simulink model "COSIM"  (R2013b)
settings: Solver=FixedStepDiscrete  StartTime=0.0  StopTime=N  RelTol=1e-3
libraries: modelsimlib x1
settings Model: Creator=o_cotte  LastModifiedBy=o_cotte

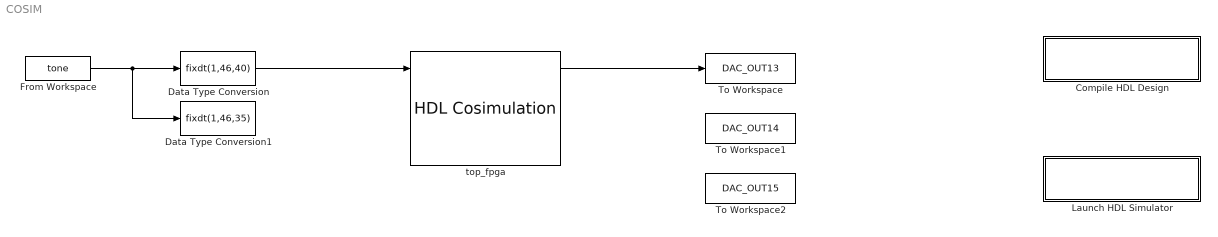
== system COSIM ==
  Compile HDL Design : Subsystem
      settings: OpenFcn=eval('compile_hdl_design_top_fpga');
      mask Display: disp(['Double-Click to' char(10) 'compile HDL files'])
  Data Type Conversion : DataTypeConversion  OutDataTypeStr=fixdt(1,46,40)
  Data Type Conversion1 : DataTypeConversion  OutDataTypeStr=fixdt(1,46,35)
  From Workspace : FromWorkspace  VariableName=tone  SampleTime=1  Interpolate=off  OutputAfterFinalValue=Cyclic repetition
  Launch HDL Simulator : Subsystem
      settings: OpenFcn=eval('launch_hdl_simulator_top_fpga');
      mask Display: disp(['Double-Click to' char(10) 'launch HDL simulator'])
  To Workspace : ToWorkspace  VariableName=DAC_OUT13  SampleTime=-1
  To Workspace1 : ToWorkspace  VariableName=DAC_OUT14  SampleTime=-1  SaveFormat=Timeseries
  To Workspace2 : ToWorkspace  VariableName=DAC_OUT15  SampleTime=-1  SaveFormat=Timeseries
  top_fpga : modelsimlib/HDL Cosimulation  PortPaths=/top_fpga/DAC_IN1;/top_fpga/DAC_IN2;/top_fpga/DAC_IN3;/top_fpga/DAC_OUT13;/top_fpga/DAC_OUT14;/top_fpga/DAC_OUT15;  PortModes=[1 1 1 2 2 2 ]  PortTimes=[-1,-1,-1,1,1,1]  PortSigns=[-1,-1,-1,1,-1,-1,]  PortFracLengths=[0,0,0,32,0,0]  CommLocal=on  CommSharedMemory=off  CommPortNumber=56757  CommShowInfo=on  ClockModes=[]  ClockTimes=[]  TclPreSimCommand=|  TclPostSimCommand=|  TimingMode=ns  TimingScaleFactor=1  idxCellArray={'UNUSED_VAR'}  CosimBypass=Full Simulation  AllowDirectFeedthrough=on  ProductName=EDA Simulator Link MQ  RunAutoTimescale=off  HdlClocks=/top_fpga/sys_clk 2.034 ns;  PreRunTime=136.278  PreRunTimeUnit=ns
      TclPreSimCommand=|
      | force /top_fpga/sys_clk 0 0 ns, 1 1.017 ns -repeat 2.034 ns;
      | force /top_fpga/sys_rst_n 0 0 ns, 1 135 ns;
      TclPostSimCommand=|
      | noforce /top_fpga/sys_clk;
      | noforce /top_fpga/sys_rst_n;
      | puts "done";
  wires:
  Data Type Conversion/1 -> top_fpga/1
  From Workspace/1 -> Data Type Conversion1/1, Data Type Conversion/1
  top_fpga/1 -> To Workspace/1

== system COSIM/Compile HDL Design ==

== system COSIM/Launch HDL Simulator ==
